simulink model "RP_DCE"  (Simulink 8.4)
settings: Solver=ode45  StartTime=0.0  StopTime=5  RelTol=1e-3
undefined symbols (not defined in the file or in its folder): Humusoft, MF614
libraries: rtlib x3
settings Model: Creator=roubalj  LastModifiedBy=Matous  ExtModeTrigMode=oneshot  ExtModeArmWhenConnect=off
settings DataIOCC: LimitDataPoints=off  SaveOutput=off
settings OptimizationCC: BlockReduction=off  BooleanDataType=off  InitFltsAndDblsToZero=on
settings DebuggingCC: SaveWithParameterizedLinksMsg=none  SignalResolutionControl=TryResolveAllWithWarning  SolverPrmCheckMsg=none  MultiTaskDSMMsg=warning  MultiTaskCondExecSysMsg=none  StrictBusMsg=None
settings HardwareCC: TargetUnknown=on
settings RTWCC: IncludeERTFirstTime=on
settings GRTTargetCC: TargetFcnLib=ansi_tfl_tmw.mat

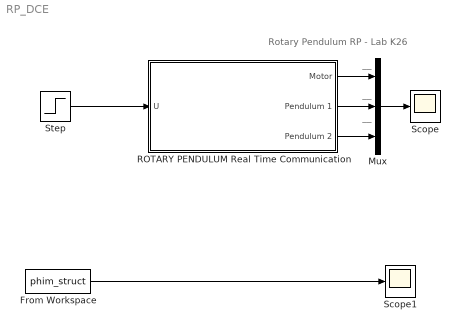
== system RP_DCE ==
  note: __
  note: __
  note: Rotary Pendulum RP - Lab K26
  note: __
  From Workspace : FromWorkspace  VariableName=phim_struct  SampleTime=0
  Mux : Mux  Inputs=3
  ROTARY PENDULUM Real Time Communication : Subsystem  mask(Rotary Pendulum RP in Laboratory K26){Ts=0.01, U_init=0, U_final=0}
      mask prompts: Ts "Sampling Time {Ts = 0.005 s; <0.02 ...0.001>}"; U_init "Initial Input Value {U_init = 0; <-1 ... 1>}"; U_final "Final Input Value {U_final = 0; <-1 ... 1>}"
      mask help: Rotary Pendulum RP in Laboratory K26 - Real Time Communication
      mask Help:
      | Rotary Pendulum in Laboratory K26 - Real Time Communication. <br><br>
      | 
      | This is a model of the Rotary Pendulum. The motor is rotate the mass with a pivot. Pendulum 1 is hung on the mass on the pivot and pendulum 2 is hugh on the pendulum 1. <br><br>
      | 
      | There are one input and three outputs in the model. The input is a volatage of the motor between -10 and 10 volts. Outputs are the real motor angle and the real angles of the pendulum 1 and pendulum 2. In Simulink, the signals are normalized to interval (-1; +1). <br><br>
      | 
      | You can set a samplig time and you can set an initial and a final value of the input voltage of the motor.
      mask Display:
      | plot(-2,-1,2,1,[-1,-1,0.3,0.3,-1],[-0.8,-0.6,-0.6,-0.8,-0.8]);
      | plot(-2,-1,2,1,[-0.8,-0.8,0,0,-0.8],[-0.6,0.8,0.8,-0.6,-0.6]);
      | plot(-2,-1,2,1,[-0.8,-0.8,0.8,0.8,-0.8],[0.6,0.8,0.8,0.6,0.6]);
      | plot(-2,-1,2,1,[-0.8,-0.6,-0.6,-0.4,-0.4,-0.2,-0.2,0,0],[0.8,0.6,0.8,0.6,0.8,0.6,0.8,0.6,0.8]);
      | plot(-2,-1,2,1,[0.7,0.8,0.8,0.7,0.7],[0.8,0.8,0.2,0.2,0.8],[0.72,0.76,0.76,0.72,0.72],[0.78,0.78,0.22,0.22,0.78],[0.74,0.72,0.72,0.74,0.74],[0.76,0.76,0.24,0.24,0.76]);
  Scope : Scope
      settings: TimeRange=5  YMin=-1000  YMax=8000  SaveName=ty  MaxDataPoints=50000
  Scope1 : Scope
      settings: TimeRange=5  YMin=-1000  YMax=8000  SaveName=ty1  MaxDataPoints=50000
  Step : Step  Before=0.2  After=0  SampleTime=0
  wires:
  ROTARY PENDULUM Real Time Communication/2(Pendulum 1) -> Mux/2
  Mux/1 -> Scope/1
  ROTARY PENDULUM Real Time Communication/1(Motor) -> Mux/1
  ROTARY PENDULUM Real Time Communication/3(Pendulum 2) -> Mux/3
  Step/1 -> ROTARY PENDULUM Real Time Communication/1(U)
  From Workspace/1 -> Scope1/1

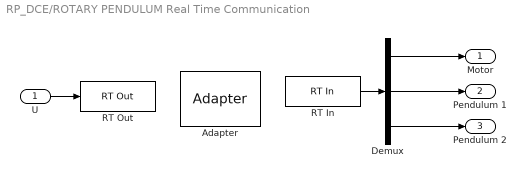
== system RP_DCE/ROTARY PENDULUM Real Time Communication ==
  U : Inport
  Adapter : rtlib/Adapter  SystemSampleTime=-1  DriverName=Humusoft/MF614  DriverAddress=4294967295  DriverOptions=0
      settings: AttributesFormatString=Humusoft\nMF614 (auto)
  Demux : Demux  Outputs=3
  RT In : rtlib/RT In  SampleTime=Ts  Adapter=Adapter  IOClass=Encoder Input  Channels=[2,4,1]  SLDataType=double  MaxMissedTicks=100  ShowMissedTicks=off  YieldWhenWaiting=on  AIORange=0 to 5 V  AIOUnits=Volts  DIOMode=Bit  CIReset=never  CIEdge=rising  CIGate=none  EIQuadrature=quadruple  EIIndexPulse=falling edge index  EIFilterFrequency=inf  OIOParameters=[]
  RT Out : rtlib/RT Out  SampleTime=Ts  Adapter=Adapter  IOClass=Analog Output  Channels=1  InitialValue=[U_init]  FinalValue=[U_final]  MaxMissedTicks=100  ShowMissedTicks=off  YieldWhenWaiting=on  AIORange=-10 to 10 V  AIOUnits=Normalized bipolar  DIOMode=Bit  OIOParameters=[]
  Motor : Outport
  Pendulum 1 : Outport  Port=2
  Pendulum 2 : Outport  Port=3
  wires:
  RT In/1 -> Demux/1
  U/1 -> RT Out/1
  Demux/3 -> Pendulum 2/1
  Demux/1 -> Motor/1
  Demux/2 -> Pendulum 1/1
